simulink model "Exc_1_4_4"  (R2021a)
settings: Solver=VariableStepAuto  StartTime=0.0  StopTime=0.20  MaxStep=1e-4  RelTol=1e-4
libraries: spsACVoltageSourceLib x2, spsCurrentMeasurementLib x1, eeGeneralControl x1, spsGroundLib x1, spsPowerLib x1, spsSeriesRLCBranchLib x1, spsRMSLib x1, spsVoltageMeasurementLib x1, spspowerguiLib x1
settings Model: Creator=up1083804  LastModifiedBy=up1083804
settings DataIOCC: ReturnWorkspaceOutputs=off

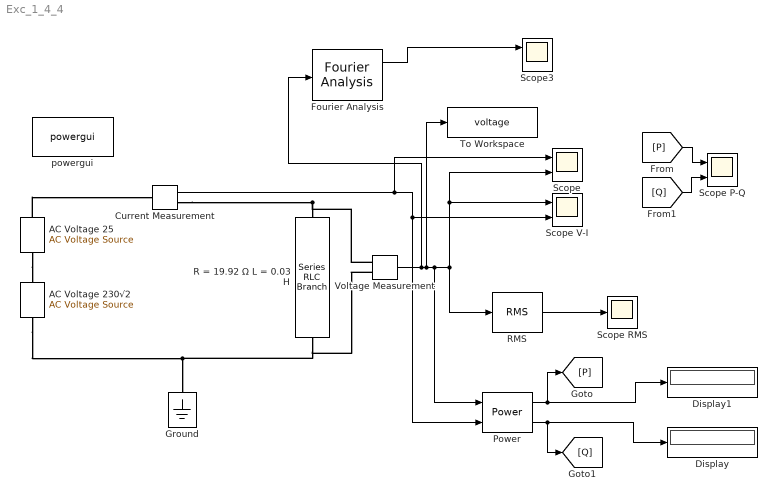
== system Exc_1_4_4 ==
  AC Voltage 230√2 : spsACVoltageSourceLib/AC Voltage Source  Amplitude=230*sqrt(2)  Phase=90  Frequency=50  SampleTime=0  Measurements=None  BusType=swing  Pref=10e3  Qref=0  Qmin=-inf  Qmax=+inf
  AC Voltage 25 : spsACVoltageSourceLib/AC Voltage Source  Amplitude=25*sqrt(2)  Phase=90  Frequency=350  SampleTime=0  Measurements=None  BusType=swing  Pref=10e3  Qref=0  Qmin=-inf  Qmax=+inf
  Current Measurement : spsCurrentMeasurementLib/Current Measurement  PhasorSimulation=off  OutputType=Complex  PSBequivalent=0
  Display : Display
  Display1 : Display
  Fourier Analysis : eeGeneralControl/Fourier Analysis  f=50  n=[1 5 7 9 ]  M0=1  Ph0=0  Ts=0
      settings: SourceProductBaseCode=PS
  Ground : spsGroundLib/Ground  LConnTagsString=a
  Power : spsPowerLib/Power  Freq=50  Vinit=[1, 0]  Iinit=[1, 0]  Ts=0
      settings: SourceProductBaseCode=PS
  R = 19.92 Ω L = 0.03 Η : spsSeriesRLCBranchLib/Series RLC Branch  LConnTagsString=__new0  RConnTagsString=__new0  BranchType=RL  Resistance=26.53  Inductance=0.049  SetiL0=off  InitialCurrent=0  Capacitance=1e-6  Setx0=off  InitialVoltage=0  Measurements=None
  RMS : spsRMSLib/RMS  TrueRMS=on  Freq=50  RMSInit=120  Ts=0
  Scope : Scope  NumInputPorts=2
  Scope P-Q : Scope  NumInputPorts=2
  Scope RMS : Scope
  Scope V-I : Scope  NumInputPorts=2
  Scope3 : Scope  NumInputPorts=2
  To Workspace : ToWorkspace  VariableName=voltage  SaveFormat=Structure With Time
  Voltage Measurement : spsVoltageMeasurementLib/Voltage Measurement  PhasorSimulation=off  OutputType=Complex  PSBequivalent=0
  powergui : spspowerguiLib/powergui  Priority=1  SimulationMode=Continuous  SampleTime=50e-6  frequency=60  Iterations=50  frequencyindice=50  Pbase=100e6  ErrMax=1e-4  UnitsV=kV  UnitsW=MW  buscounter=0  FunctionMessages=off  echomessages=off  EnableUseOfTLC=off  CurrentSourceSwitches=off  DisableSnubberDevices=off  DisableRonSwitches=off  DisableVfSwitches=off  DisplayEquations=off  AutomaticDiscreteSolvers=off  SolverType=Tustin/Backward Euler (TBE)  Interpol=off  ExternalGateDelay=off  methode=off  Ts=100  x0status=blocks  SPID=on  SwTol=0  HookPort=off  NonlinearTolerance=1e-4  nMaxIteration=100  ContinueOnMaxIteration=off  RestoreLinks=warning  ResistiveCurrentMeasurement=off  Frange=[0:2:500]  Ylog=off  Xlog=on  ShowGrid=off  save=off  variable=ZData  structure=0  ZoomFFT=off  StartTime=0.0  cycles=1  DisplayStyle=1  fundamental=60  FreqAxis=off  MaxFrequency=1000  frequencyindicesteady=1  RmsSteady=1  display=off
  wires:
  Current Measurement/1 -> Scope/1, Power/2, Scope V-I/2
  RMS/1 -> Scope RMS/1
  Voltage Measurement/1 -> To Workspace/1, Power/1, RMS/1, Scope/2, Scope V-I/1, Fourier Analysis/1
  Fourier Analysis/1 -> Scope3/1
  [P] -> Scope P-Q/1
  Power/2 -> [Q], Display/1
  Power/1 -> Display1/1, [P]
  [Q] -> Scope P-Q/2
  connections:
  AC Voltage 230√2/LConn1 -- Voltage Measurement/LConn2 -- R = 19.92 Ω L = 0.03 Η/RConn1 -- Ground/LConn1
  Current Measurement/RConn1 -- Voltage Measurement/LConn1 -- R = 19.92 Ω L = 0.03 Η/LConn1
  AC Voltage 25/LConn1 -- AC Voltage 230√2/RConn1
  AC Voltage 25/RConn1 -- Current Measurement/LConn1
